simulink model "Control_I_PD"  (R2021a)
settings: Solver=VariableStepAuto  StartTime=0.0  StopTime=10.0  RelTol=1e-3
values from neighbouring files (symbols this model uses):
  A_bar = Co_inv*A*Co    [control.m]
  B_bar = Co_inv*B    [control.m]
  K1 = K(1)    [control.m]
  K2 = K(2)    [control.m]
undefined symbols (not defined in the file or in its folder): C, D
settings Model: Creator=dherr  LastModifiedBy=dherr
settings DataIOCC: SaveOutput=off  ReturnWorkspaceOutputs=off

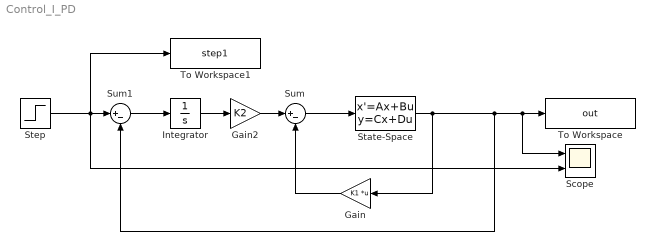
== system Control_I_PD ==
  Gain : Gain  Gain=K1  Multiplication=Matrix(K*u)
  Gain2 : Gain  Gain=K2
  Integrator : Integrator
  Scope : Scope  NumInputPorts=2
  State-Space : StateSpace  A=A_bar  B=B_bar  C=C  D=D  InitialCondition=0
  Step : Step  SampleTime=0
  Sum : Sum  Inputs=|+-
  Sum1 : Sum  Inputs=|+-
  To Workspace : ToWorkspace  VariableName=out  SaveFormat=Structure With Time  SampleTime=-1
  To Workspace1 : ToWorkspace  VariableName=step1  SaveFormat=Structure With Time  SampleTime=-1
  wires:
  Sum1/1 -> Integrator/1
  Integrator/1 -> Gain2/1
  Step/1 -> Scope/2, Sum1/1, To Workspace1/1
  Sum/1 -> State-Space/1
  Gain2/1 -> Sum/1
  Gain/1 -> Sum/2
  State-Space/1 -> Sum1/2, Scope/1, To Workspace/1, Gain/1
